simulink model "Q3_Composite"  (R2026a)
settings: Solver=ode45  StopTime=5  RelTol=1e-8  AbsTol=1e-10
model workspace (MAT data in the model file):
  input_signal = timeseries
  input_signal.Name = 'unnamed'
  input_signal.DataInfo = tsdata.datametadata
  input_signal.DataInfo.Interpolation = tsdata.interpolation
  input_signal.DataInfo.Interpolation.Fhandle : function handle (value not decoded)
  input_signal.DataInfo.Interpolation.Name = 'linear'
  input_signal.TimeInfo = tsdata.timemetadata
  input_signal.TimeInfo.Length = 2501
  input_signal.TimeInfo.DuplicateTimes = 0
  input_signal.TimeInfo.Time_ = [0 0.002 0.004 0.006 0.008 0.01 0.012 0.014 0.016 0.018 0.02 0.022 ... (2501 elements, 2501x1)]
  input_signal.TimeInfo.Initialized = 1
  input_signal.QualityInfo = tsdata.qualmetadata
  input_signal.Data_ = [2 1.99401596405 1.98806371287 1.98214303241 1.97625370993 1.97039553397 1.96456829435 1.95877178217 1.95300578981 1.94727011088 1.94156454025 1.93588887405 ... (2501 elements, 2501x1)]
settings Model: Creator=szj  LastModifiedBy=szj

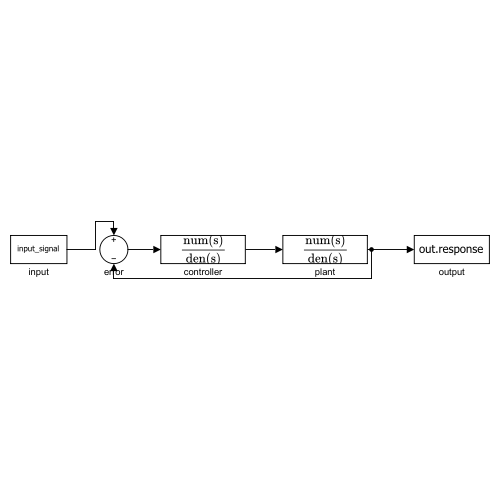
[thumbnail: Simulink's stored preview of the top-level diagram]
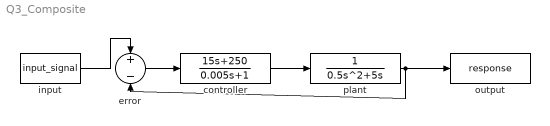
== system Q3_Composite ==
  controller : TransferFcn  Numerator=[15 250]  Denominator=[0.005 1]
  error : Sum  Inputs=+-
  input : FromWorkspace  VariableName=input_signal
  output : ToWorkspace  VariableName=response  SaveFormat=Timeseries  SampleTime=-1
  plant : TransferFcn  Numerator=[0 0 1]  Denominator=[0.5 5 0]
  wires:
  input/1 -> error/1
  error/1 -> controller/1
  controller/1 -> plant/1
  plant/1 -> output/1, error/2
